simulink model "type2_STC"  (R2024b)
settings: Solver=VariableStepAuto  StartTime=0.0  StopTime=10.0  RelTol=1e-3
libraries: simulink x3
(part 2 of 2)

== system type2_STC/Subsystem/Subsystem3/Subsystem7 ==
  In1 : Inport
  Constant1 : Constant
  Constant2 : Constant  Value=0
  Switch6 : Switch  Criteria=u2 > Threshold  Threshold=3  SaturateOnIntegerOverflow=off  InputSameDT=off
  Out1 : Outport
  wires:
  Constant2/1 -> Switch6/3
  Switch6/1 -> Out1/1
  Constant1/1 -> Switch6/1
  In1/1 -> Switch6/2

== system type2_STC/Subsystem/Subsystem8/Subsystem2 ==
  In1 : Inport
  Constant1 : Constant
  Constant2 : Constant  Value=0
  Switch6 : Switch  Criteria=u2 > Threshold  Threshold=3  SaturateOnIntegerOverflow=off  InputSameDT=off
  Out1 : Outport
  wires:
  Constant2/1 -> Switch6/3
  Switch6/1 -> Out1/1
  Constant1/1 -> Switch6/1
  In1/1 -> Switch6/2

== system type2_STC/Subsystem/Subsystem8/Subsystem3 ==
  In1 : Inport
  Constant3 : Constant  Value=0
  Switch10 : Switch  Criteria=u2 > Threshold  Threshold=3  SaturateOnIntegerOverflow=off  InputSameDT=off
  Out1 : Outport
  wires:
  In1/1 -> Switch10/2, Switch10/3
  Constant3/1 -> Switch10/1
  Switch10/1 -> Out1/1

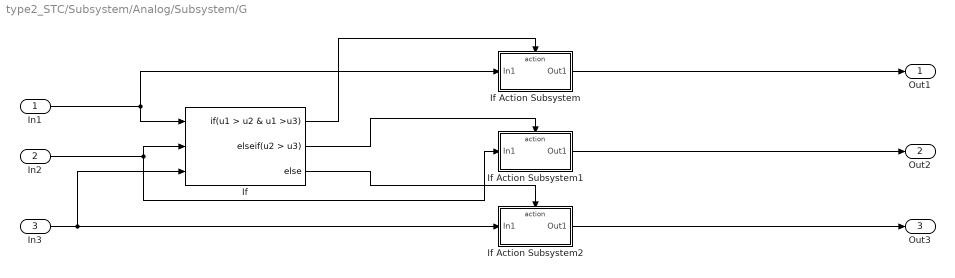
== system type2_STC/Subsystem/Analog/Subsystem/G ==
  In1 : Inport
  In2 : Inport  Port=2
  In3 : Inport  Port=3
  If : If  NumInputs=3  IfExpression=u1 > u2 & u1 >u3  ElseIfExpressions=u2 > u3
  If Action Subsystem : Subsystem  TreatAsAtomicUnit=on
  If Action Subsystem1 : Subsystem  TreatAsAtomicUnit=on
  If Action Subsystem2 : Subsystem  TreatAsAtomicUnit=on
  Out1 : Outport
  Out2 : Outport  Port=2
  Out3 : Outport  Port=3
  wires:
  If/3 -> If Action Subsystem2/Action
  If/1 -> If Action Subsystem/Action
  In2/1 -> If Action Subsystem1/1(In1), If/2
  In1/1 -> If Action Subsystem/1(In1), If/1
  If/2 -> If Action Subsystem1/Action
  In3/1 -> If/3, If Action Subsystem2/1(In1)
  If Action Subsystem1/1(Out1) -> Out2/1
  If Action Subsystem/1(Out1) -> Out1/1
  If Action Subsystem2/1(Out1) -> Out3/1

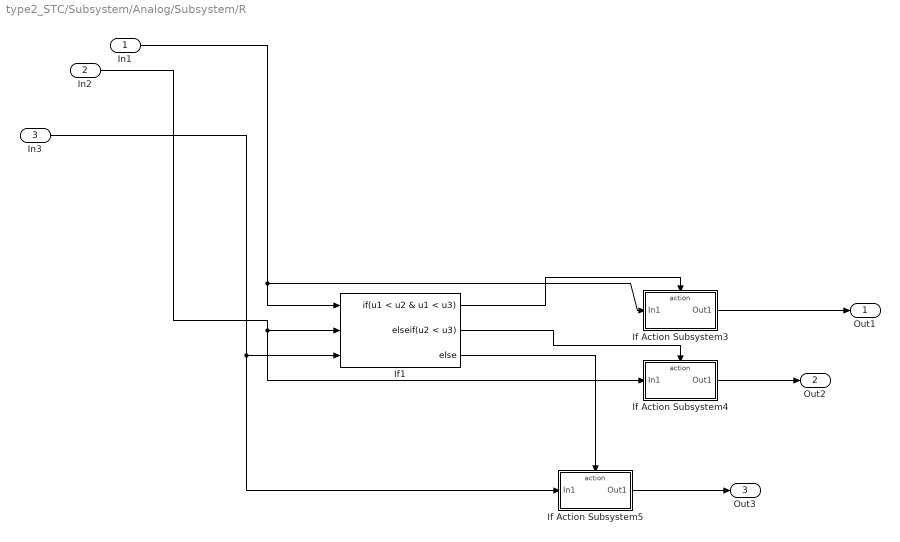
== system type2_STC/Subsystem/Analog/Subsystem/R ==
  In1 : Inport
  In2 : Inport  Port=2
  In3 : Inport  Port=3
  If Action Subsystem3 : Subsystem  TreatAsAtomicUnit=on
  If Action Subsystem4 : Subsystem  TreatAsAtomicUnit=on
  If Action Subsystem5 : Subsystem  TreatAsAtomicUnit=on
  If1 : If  NumInputs=3  IfExpression=u1 < u2 & u1 < u3  ElseIfExpressions=u2 < u3
  Out1 : Outport
  Out2 : Outport  Port=2
  Out3 : Outport  Port=3
  wires:
  If1/2 -> If Action Subsystem4/Action
  In3/1 -> If Action Subsystem5/1(In1), If1/3
  If Action Subsystem3/1(Out1) -> Out1/1
  In1/1 -> If1/1, If Action Subsystem3/1(In1)
  In2/1 -> If Action Subsystem4/1(In1), If1/2
  If1/1 -> If Action Subsystem3/Action
  If Action Subsystem4/1(Out1) -> Out2/1
  If1/3 -> If Action Subsystem5/Action
  If Action Subsystem5/1(Out1) -> Out3/1

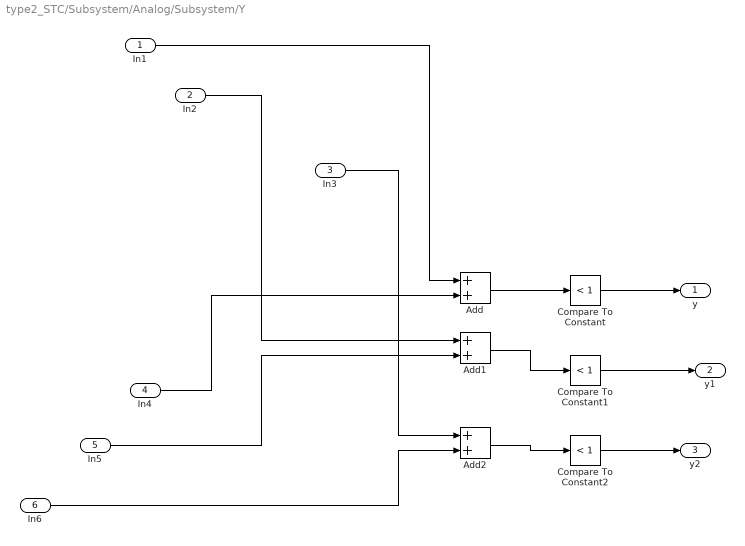
== system type2_STC/Subsystem/Analog/Subsystem/Y ==
  In1 : Inport
  In2 : Inport  Port=2
  In3 : Inport  Port=3
  In4 : Inport  Port=4
  In5 : Inport  Port=5
  In6 : Inport  Port=6
  Add : Sum
  Add1 : Sum
  Add2 : Sum
  Compare To Constant : simulink/Logic and Bit Operations/Compare To Constant  relop=<  const=1  OutDataTypeStr=boolean
  Compare To Constant1 : simulink/Logic and Bit Operations/Compare To Constant  relop=<  const=1  OutDataTypeStr=boolean
  Compare To Constant2 : simulink/Logic and Bit Operations/Compare To Constant  relop=<  const=1  OutDataTypeStr=boolean
  y : Outport
  y1 : Outport  Port=2
  y2 : Outport  Port=3
  wires:
  Add/1 -> Compare To Constant/1
  In2/1 -> Add1/1
  Compare To Constant1/1 -> y1/1
  In4/1 -> Add/2
  Compare To Constant/1 -> y/1
  Add1/1 -> Compare To Constant1/1
  Add2/1 -> Compare To Constant2/1
  In5/1 -> Add1/2
  In3/1 -> Add2/1
  In1/1 -> Add/1
  In6/1 -> Add2/2
  Compare To Constant2/1 -> y2/1

== system type2_STC/Subsystem/Analog/Subsystem/G/If Action Subsystem ==
  In1 : Inport
  Action Port : ActionPort  ActionPortLabel=if(u1 > u2 & u1 >u3)
  Constant : Constant
  Constant1 : Constant  Value=3
  Display : Display
  Switch : Switch  Threshold=1  SaturateOnIntegerOverflow=off  InputSameDT=off
  Out1 : Outport
  wires:
  In1/1 -> Switch/2
  Constant1/1 -> Switch/1
  Constant/1 -> Switch/3
  Switch/1 -> Display/1, Out1/1

== system type2_STC/Subsystem/Analog/Subsystem/G/If Action Subsystem1 ==
  In1 : Inport
  Action Port : ActionPort  ActionPortLabel=elseif(u2 > u3)
  Constant : Constant  Value=3
  Constant1 : Constant
  Switch : Switch  Threshold=1  SaturateOnIntegerOverflow=off  InputSameDT=off
  Out1 : Outport
  wires:
  In1/1 -> Switch/2
  Constant/1 -> Switch/1
  Constant1/1 -> Switch/3
  Switch/1 -> Out1/1

== system type2_STC/Subsystem/Analog/Subsystem/G/If Action Subsystem2 ==
  In1 : Inport
  Action Port : ActionPort  ActionPortLabel=else
  Constant : Constant  Value=3
  Constant1 : Constant
  Switch : Switch  Threshold=1  SaturateOnIntegerOverflow=off  InputSameDT=off
  Out1 : Outport
  wires:
  In1/1 -> Switch/2
  Constant/1 -> Switch/1
  Constant1/1 -> Switch/3
  Switch/1 -> Out1/1

== system type2_STC/Subsystem/Analog/Subsystem/R/If Action Subsystem3 ==
  In1 : Inport
  Action Port : ActionPort  ActionPortLabel=if(u1 < u2 & u1 < u3)
  Constant : Constant  Value=2
  Constant1 : Constant  Value=0
  Switch : Switch  SaturateOnIntegerOverflow=off  InputSameDT=off
  Out1 : Outport
  wires:
  Constant1/1 -> Switch/3
  In1/1 -> Switch/2
  Constant/1 -> Switch/1
  Switch/1 -> Out1/1

== system type2_STC/Subsystem/Analog/Subsystem/R/If Action Subsystem4 ==
  In1 : Inport
  Action Port : ActionPort  ActionPortLabel=elseif(u2 < u3)
  Constant : Constant  Value=2
  Constant1 : Constant  Value=0
  Switch : Switch  SaturateOnIntegerOverflow=off  InputSameDT=off
  Out1 : Outport
  wires:
  Constant1/1 -> Switch/3
  In1/1 -> Switch/2
  Constant/1 -> Switch/1
  Switch/1 -> Out1/1

== system type2_STC/Subsystem/Analog/Subsystem/R/If Action Subsystem5 ==
  In1 : Inport
  Action Port : ActionPort  ActionPortLabel=else
  Constant : Constant  Value=2
  Constant1 : Constant  Value=0
  Switch : Switch  SaturateOnIntegerOverflow=off  InputSameDT=off
  Out1 : Outport
  wires:
  In1/1 -> Switch/2
  Constant/1 -> Switch/1
  Constant1/1 -> Switch/3
  Switch/1 -> Out1/1
